simulink model "mat_model"  (R2013b)
settings: Solver=ode3  StartTime=0.0  StopTime=0.06  FixedStep=100e-6  RelTol=1e-3
undefined symbols (not defined in the file): E, f, L, L1, R, Ts
settings Model: Creator=sadzi  LastModifiedBy=sadzi
settings SolverCC: AlgebraicLoopSolver=LineSearch
settings ConfigurationSet: Description=SimMechanics 2G

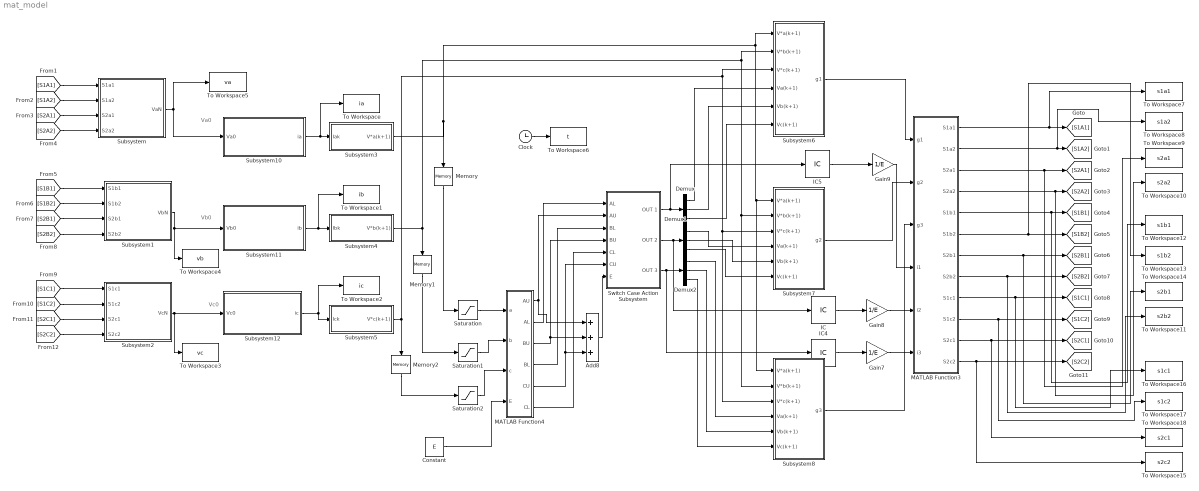
== system mat_model ==
  note: Vc0
  note: Va0
  note: Vb0
  Add8 : Sum  Inputs=+++
  Clock : Clock
  Constant : Constant  Value=E
  Demux : Demux  Outputs=3
  Demux1 : Demux  Outputs=3
  Demux2 : Demux  Outputs=3
  Gain7 : Gain  Gain=1/E
  Gain8 : Gain  Gain=1/E
  Gain9 : Gain  Gain=1/E
  IC : InitialCondition  Value=[0 0 0]
  IC4 : InitialCondition  Value=[0 0 0]
  IC5 : InitialCondition  Value=[0 0 0]
  MATLAB Function3 : MATLAB Function  TreatAsAtomicUnit=on
  MATLAB Function4 : MATLAB Function  TreatAsAtomicUnit=on
  Memory : Memory
  Memory1 : Memory
  Memory2 : Memory
  Saturation : Saturate  UpperLimit=2*E  LowerLimit=-2*E
  Saturation1 : Saturate  UpperLimit=2*E  LowerLimit=-2*E
  Saturation2 : Saturate  UpperLimit=2*E  LowerLimit=-2*E
  Subsystem : Subsystem
  Subsystem1 : Subsystem
  Subsystem10 : Subsystem
  Subsystem11 : Subsystem
  Subsystem12 : Subsystem
  Subsystem2 : Subsystem
  Subsystem3 : Subsystem
  Subsystem4 : Subsystem
  Subsystem5 : Subsystem
  Subsystem6 : Subsystem
  Subsystem7 : Subsystem
  Subsystem8 : Subsystem
  Switch Case Action Subsystem : Subsystem  TreatAsAtomicUnit=on
  To Workspace : ToWorkspace  VariableName=ia  SampleTime=-1
  To Workspace1 : ToWorkspace  VariableName=ib  SampleTime=-1
  To Workspace10 : ToWorkspace  VariableName=s2a2  SampleTime=-1
  To Workspace11 : ToWorkspace  VariableName=s2b2  SampleTime=-1
  To Workspace12 : ToWorkspace  VariableName=s1b1  SampleTime=-1
  To Workspace13 : ToWorkspace  VariableName=s1b2  SampleTime=-1
  To Workspace14 : ToWorkspace  VariableName=s2b1  SampleTime=-1
  To Workspace15 : ToWorkspace  VariableName=s2c2  SampleTime=-1
  To Workspace16 : ToWorkspace  VariableName=s1c1  SampleTime=-1
  To Workspace17 : ToWorkspace  VariableName=s1c2  SampleTime=-1
  To Workspace18 : ToWorkspace  VariableName=s2c1  SampleTime=-1
  To Workspace2 : ToWorkspace  VariableName=ic  SampleTime=-1
  To Workspace3 : ToWorkspace  VariableName=vc  SampleTime=-1
  To Workspace4 : ToWorkspace  VariableName=vb  SampleTime=-1
  To Workspace5 : ToWorkspace  VariableName=va  SampleTime=-1
  To Workspace6 : ToWorkspace  VariableName=t  SampleTime=-1
  To Workspace7 : ToWorkspace  VariableName=s1a1  SampleTime=-1
  To Workspace8 : ToWorkspace  VariableName=s1a2  SampleTime=-1
  To Workspace9 : ToWorkspace  VariableName=s2a1  SampleTime=-1
  wires:
  Subsystem/1(VaN) -> To Workspace5/1, Subsystem10/1(Va0)
  Subsystem3/1(V*a(k+1)) -> Subsystem8/1(V*a(k+1)), Subsystem7/1(V*a(k+1)), Subsystem6/1(V*a(k+1)), Memory/1
  Subsystem4/1(V*b(k+1)) -> Subsystem8/2(V*b(k+1)), Subsystem7/2(V*b(k+1)), Subsystem6/2(V*b(k+1)), Memory1/1
  Subsystem5/1(V*c(k+1)) -> Subsystem8/3(V*c(k+1)), Subsystem7/3(V*c(k+1)), Subsystem6/3(V*c(k+1)), Memory2/1
  MATLAB Function4/1(AU) -> Add8/1, Switch Case Action Subsystem/2(AU)
  MATLAB Function4/3(BU) -> Add8/2, Switch Case Action Subsystem/4(BU)
  MATLAB Function4/5(CU) -> Add8/3, Switch Case Action Subsystem/6(CU)
  MATLAB Function4/2(AL) -> Switch Case Action Subsystem/1(AL)
  MATLAB Function4/4(BL) -> Switch Case Action Subsystem/3(BL)
  MATLAB Function4/6(CL) -> Switch Case Action Subsystem/5(CL)
  Switch Case Action Subsystem/1(OUT 1) -> Demux/1, IC5/1
  Demux/1 -> Subsystem6/4(Va(k+1))
  Demux/2 -> Subsystem6/5(Vb(k+1))
  Demux/3 -> Subsystem6/6(Vc(k+1))
  Switch Case Action Subsystem/2(OUT 2) -> IC/1, Demux1/1
  Demux1/1 -> Subsystem7/4(Va(k+1))
  Demux1/2 -> Subsystem7/5(Vb(k+1))
  Demux1/3 -> Subsystem7/6(Vc(k+1))
  Switch Case Action Subsystem/3(OUT 3) -> IC4/1, Demux2/1
  Demux2/1 -> Subsystem8/4(Va(k+1))
  Demux2/2 -> Subsystem8/5(Vb(k+1))
  Demux2/3 -> Subsystem8/6(Vc(k+1))
  Subsystem1/1(VbN) -> To Workspace4/1, Subsystem11/1(Vb0)
  Subsystem2/1(VcN) -> To Workspace3/1, Subsystem12/1(Vc0)
  Subsystem7/1(g2) -> MATLAB Function3/2(g2)
  Subsystem6/1(g1) -> MATLAB Function3/1(g1)
  Subsystem8/1(g3) -> MATLAB Function3/3(g3)
  Saturation/1 -> MATLAB Function4/1(a)
  Saturation1/1 -> MATLAB Function4/2(b)
  Saturation2/1 -> MATLAB Function4/3(c)
  Add8/1 -> Switch Case Action Subsystem/7(E)
  Gain7/1 -> MATLAB Function3/6(i3)
  Gain8/1 -> MATLAB Function3/5(i2)
  Gain9/1 -> MATLAB Function3/4(i1)
  [S1A2] -> Subsystem/2(S1a2)
  [S2A1] -> Subsystem/3(S2a1)
  [S2A2] -> Subsystem/4(S2a2)
  [S1B1] -> Subsystem1/1(S1b1)
  [S1B2] -> Subsystem1/2(S1b2)
  [S2B1] -> Subsystem1/3(S2b1)
  [S2B2] -> Subsystem1/4(S2b2)
  [S1C1] -> Subsystem2/1(S1c1)
  [S1C2] -> Subsystem2/2(S1c2)
  [S2C1] -> Subsystem2/3(S2c1)
  [S2C2] -> Subsystem2/4(S2c2)
  [S1A1] -> Subsystem/1(S1a1)
  MATLAB Function3/1(S1a1) -> To Workspace7/1, [S1A1]
  IC/1 -> Gain8/1
  IC4/1 -> Gain7/1
  IC5/1 -> Gain9/1
  MATLAB Function3/2(S1a2) -> To Workspace8/1, [S1A2]
  MATLAB Function3/3(S2a1) -> To Workspace9/1, [S2A1]
  MATLAB Function3/4(S2a2) -> To Workspace10/1, [S2A2]
  MATLAB Function3/5(S1b1) -> To Workspace12/1, [S1B1]
  MATLAB Function3/6(S1b2) -> To Workspace13/1, [S1B2]
  MATLAB Function3/7(S2b1) -> To Workspace14/1, [S2B1]
  MATLAB Function3/8(S2b2) -> To Workspace11/1, [S2B2]
  MATLAB Function3/9(S1c1) -> To Workspace16/1, [S1C1]
  MATLAB Function3/10(S1c2) -> To Workspace17/1, [S1C2]
  MATLAB Function3/11(S2c1) -> To Workspace18/1, [S2C1]
  MATLAB Function3/12(S2c2) -> To Workspace15/1, [S2C2]
  Memory/1 -> Saturation/1
  Memory1/1 -> Saturation1/1
  Memory2/1 -> Saturation2/1
  Constant/1 -> MATLAB Function4/4(E)
  Subsystem10/1(ia) -> To Workspace/1, Subsystem3/1(Iak)
  Subsystem11/1(ib) -> To Workspace1/1, Subsystem4/1(Ibk)
  Subsystem12/1(ic) -> To Workspace2/1, Subsystem5/1(Ick)
  Clock/1 -> To Workspace6/1

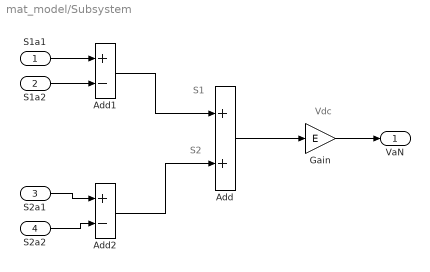
== system mat_model/Subsystem ==
  note: Vdc
  note: S2
  note: S1
  S1a1 : Inport
  S1a2 : Inport  Port=2
  S2a1 : Inport  Port=3
  S2a2 : Inport  Port=4
  Add : Sum
  Add1 : Sum  Inputs=+-
  Add2 : Sum  Inputs=+-
  Gain : Gain  Gain=E
  VaN : Outport
  wires:
  Add2/1 -> Add/2
  Add1/1 -> Add/1
  Add/1 -> Gain/1
  Gain/1 -> VaN/1
  S1a1/1 -> Add1/1
  S1a2/1 -> Add1/2
  S2a1/1 -> Add2/1
  S2a2/1 -> Add2/2

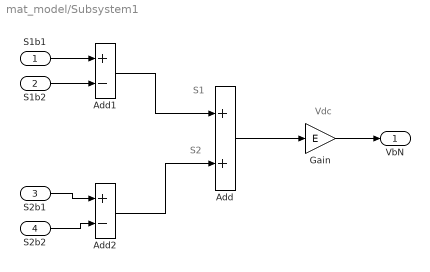
== system mat_model/Subsystem1 ==
  note: Vdc
  note: S2
  note: S1
  S1b1 : Inport
  S1b2 : Inport  Port=2
  S2b1 : Inport  Port=3
  S2b2 : Inport  Port=4
  Add : Sum
  Add1 : Sum  Inputs=+-
  Add2 : Sum  Inputs=+-
  Gain : Gain  Gain=E
  VbN : Outport
  wires:
  Add2/1 -> Add/2
  Add1/1 -> Add/1
  Add/1 -> Gain/1
  Gain/1 -> VbN/1
  S1b1/1 -> Add1/1
  S1b2/1 -> Add1/2
  S2b1/1 -> Add2/1
  S2b2/1 -> Add2/2

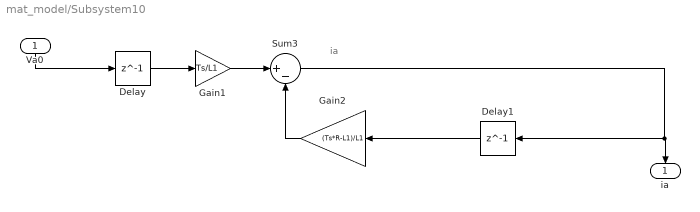
== system mat_model/Subsystem10 ==
  note: ia
  Va0 : Inport
  Delay : Delay  DelayLength=1  InitialCondition=0
  Delay1 : Delay  DelayLength=1  InitialCondition=0
  Gain1 : Gain  Gain=Ts/L1
  Gain2 : Gain  Gain=(Ts*R-L1)/L1
  Sum3 : Sum  Inputs=|+-
  ia : Outport
  wires:
  Delay/1 -> Gain1/1
  Gain1/1 -> Sum3/1
  Sum3/1 -> ia/1, Delay1/1
  Delay1/1 -> Gain2/1
  Gain2/1 -> Sum3/2
  Va0/1 -> Delay/1

== system mat_model/Subsystem11 ==
  note: ib
  Vb0 : Inport
  Delay2 : Delay  DelayLength=1  InitialCondition=0
  Delay3 : Delay  DelayLength=1  InitialCondition=0
  Gain3 : Gain  Gain=Ts/L
  Gain4 : Gain  Gain=(Ts*R-L)/L
  Sum1 : Sum  Inputs=|+-
  ib : Outport
  wires:
  Vb0/1 -> Delay2/1
  Delay2/1 -> Gain3/1
  Sum1/1 -> ib/1, Delay3/1
  Gain4/1 -> Sum1/2
  Gain3/1 -> Sum1/1
  Delay3/1 -> Gain4/1

== system mat_model/Subsystem12 ==
  note: ic
  Vc0 : Inport
  Delay4 : Delay  DelayLength=1  InitialCondition=0
  Delay5 : Delay  DelayLength=1  InitialCondition=0
  Gain5 : Gain  Gain=Ts/L
  Gain6 : Gain  Gain=(Ts*R-L)/L
  Sum2 : Sum  Inputs=|+-
  ic : Outport
  wires:
  Vc0/1 -> Delay4/1
  Delay4/1 -> Gain5/1
  Gain5/1 -> Sum2/1
  Delay5/1 -> Gain6/1
  Sum2/1 -> ic/1, Delay5/1
  Gain6/1 -> Sum2/2

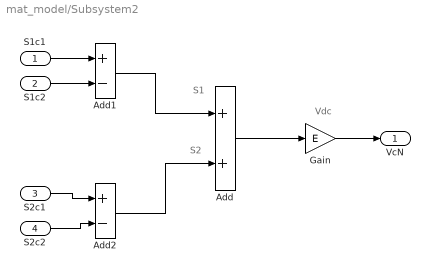
== system mat_model/Subsystem2 ==
  note: Vdc
  note: S2
  note: S1
  S1c1 : Inport
  S1c2 : Inport  Port=2
  S2c1 : Inport  Port=3
  S2c2 : Inport  Port=4
  Add : Sum
  Add1 : Sum  Inputs=+-
  Add2 : Sum  Inputs=+-
  Gain : Gain  Gain=E
  VcN : Outport
  wires:
  Add2/1 -> Add/2
  Add1/1 -> Add/1
  Add/1 -> Gain/1
  Gain/1 -> VcN/1
  S1c1/1 -> Add1/1
  S1c2/1 -> Add1/2
  S2c1/1 -> Add2/1
  S2c2/1 -> Add2/2

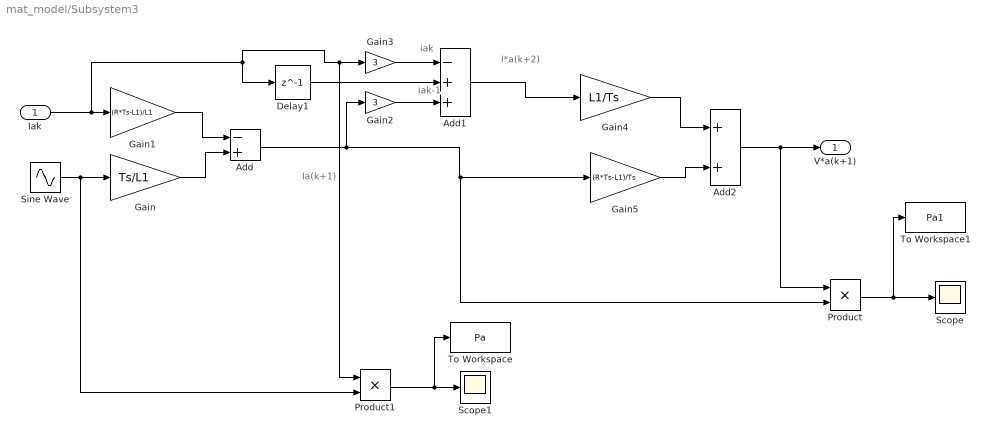
== system mat_model/Subsystem3 ==
  note: iak
  note: iak-1
  note: I*a(k+2)
  note: Ia(k+1)
  Iak : Inport
  Add : Sum  Inputs=-+
  Add1 : Sum  Inputs=-++
  Add2 : Sum
  Delay1 : Delay  DelayLength=1  InitialCondition=0
  Gain : Gain  Gain=Ts/L1
  Gain1 : Gain  Gain=(R*Ts-L1)/L1
  Gain2 : Gain  Gain=3
  Gain3 : Gain  Gain=3
  Gain4 : Gain  Gain=L1/Ts
  Gain5 : Gain  Gain=(R*Ts-L1)/Ts
  Product : Product
  Product1 : Product
  Scope : Scope
  Scope1 : Scope
  Sine Wave : Sin  SineType=Sample based  Amplitude=2*E  Frequency=f  Samples=spp  SampleTime=Ts
  To Workspace : ToWorkspace  VariableName=Pa  SampleTime=-1
  To Workspace1 : ToWorkspace  VariableName=Pa1  SampleTime=-1
  V*a(k+1) : Outport
  wires:
  Gain/1 -> Add/2
  Gain1/1 -> Add/1
  Add/1 -> Gain2/1, Product/2, Gain5/1
  Gain3/1 -> Add1/1
  Gain2/1 -> Add1/3
  Add1/1 -> Gain4/1
  Gain4/1 -> Add2/1
  Gain5/1 -> Add2/2
  Add2/1 -> Product/1, V*a(k+1)/1
  Sine Wave/1 -> Product1/2, Gain/1
  Delay1/1 -> Add1/2
  Product/1 -> To Workspace1/1, Scope/1
  Product1/1 -> To Workspace/1, Scope1/1
  Iak/1 -> Delay1/1, Product1/1, Gain3/1, Gain1/1

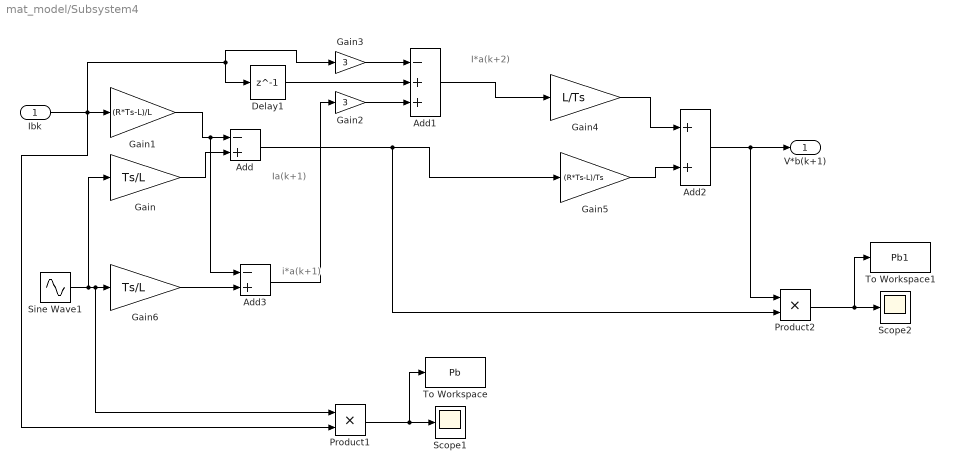
== system mat_model/Subsystem4 ==
  note: Ia(k+1)
  note: I*a(k+2)
  note: i*a(k+1)
  Ibk : Inport
  Add : Sum  Inputs=-+
  Add1 : Sum  Inputs=-++
  Add2 : Sum
  Add3 : Sum  Inputs=-+
  Delay1 : Delay  DelayLength=1  InitialCondition=0
  Gain : Gain  Gain=Ts/L
  Gain1 : Gain  Gain=(R*Ts-L)/L
  Gain2 : Gain  Gain=3
  Gain3 : Gain  Gain=3
  Gain4 : Gain  Gain=L/Ts
  Gain5 : Gain  Gain=(R*Ts-L)/Ts
  Gain6 : Gain  Gain=Ts/L
  Product1 : Product
  Product2 : Product
  Scope1 : Scope
      settings: SaveName=ScopeData2
  Scope2 : Scope
      settings: SaveName=ScopeData3
  Sine Wave1 : Sin  SineType=Sample based  Amplitude=2*E  Frequency=f  Phase=2.0943951  Samples=spp  SampleTime=Ts  Offset=nofs1
  To Workspace : ToWorkspace  VariableName=Pb  SampleTime=-1
  To Workspace1 : ToWorkspace  VariableName=Pb1  SampleTime=-1
  V*b(k+1) : Outport
  wires:
  Add2/1 -> Product2/1, V*b(k+1)/1
  Gain5/1 -> Add2/2
  Gain4/1 -> Add2/1
  Add1/1 -> Gain4/1
  Gain2/1 -> Add1/3
  Gain3/1 -> Add1/1
  Add/1 -> Product2/2, Gain5/1
  Gain/1 -> Add/2
  Sine Wave1/1 -> Gain/1, Product1/1, Gain6/1
  Gain1/1 -> Add3/1, Add/1
  Gain6/1 -> Add3/2
  Add3/1 -> Gain2/1
  Delay1/1 -> Add1/2
  Ibk/1 -> Gain3/1, Delay1/1, Product1/2, Gain1/1
  Product1/1 -> To Workspace/1, Scope1/1
  Product2/1 -> To Workspace1/1, Scope2/1

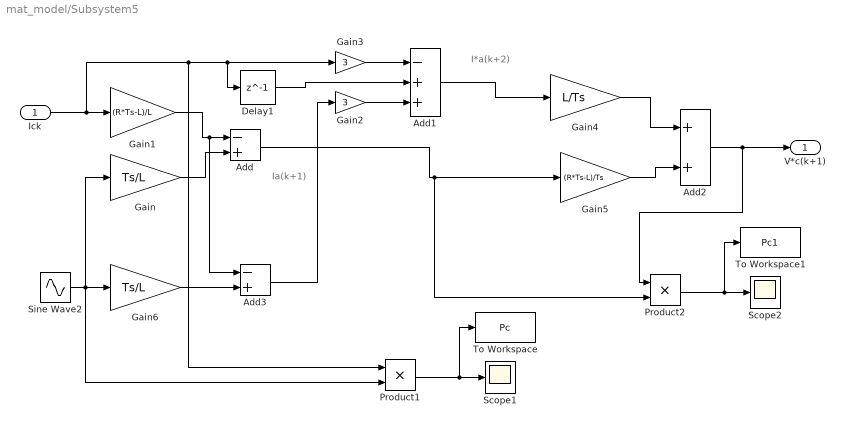
== system mat_model/Subsystem5 ==
  note: I*a(k+2)
  note: Ia(k+1)
  Ick : Inport
  Add : Sum  Inputs=-+
  Add1 : Sum  Inputs=-++
  Add2 : Sum
  Add3 : Sum  Inputs=-+
  Delay1 : Delay  DelayLength=1  InitialCondition=0
  Gain : Gain  Gain=Ts/L
  Gain1 : Gain  Gain=(R*Ts-L)/L
  Gain2 : Gain  Gain=3
  Gain3 : Gain  Gain=3
  Gain4 : Gain  Gain=L/Ts
  Gain5 : Gain  Gain=(R*Ts-L)/Ts
  Gain6 : Gain  Gain=Ts/L
  Product1 : Product
  Product2 : Product
  Scope1 : Scope
      settings: SaveName=ScopeData4
  Scope2 : Scope
      settings: SaveName=ScopeData5
  Sine Wave2 : Sin  SineType=Sample based  Amplitude=2*E  Frequency=f  Phase=4.1887902  Samples=spp  SampleTime=Ts  Offset=nofs2
  To Workspace : ToWorkspace  VariableName=Pc  SampleTime=-1
  To Workspace1 : ToWorkspace  VariableName=Pc1  SampleTime=-1
  V*c(k+1) : Outport
  wires:
  Gain/1 -> Add/2
  Add/1 -> Product2/2, Gain5/1
  Gain3/1 -> Add1/1
  Gain2/1 -> Add1/3
  Add1/1 -> Gain4/1
  Gain4/1 -> Add2/1
  Gain5/1 -> Add2/2
  Add2/1 -> Product2/1, V*c(k+1)/1
  Sine Wave2/1 -> Product1/2, Gain/1, Gain6/1
  Gain1/1 -> Add3/1, Add/1
  Gain6/1 -> Add3/2
  Add3/1 -> Gain2/1
  Delay1/1 -> Add1/2
  Ick/1 -> Product1/1, Delay1/1, Gain3/1, Gain1/1
  Product1/1 -> To Workspace/1, Scope1/1
  Product2/1 -> To Workspace1/1, Scope2/1

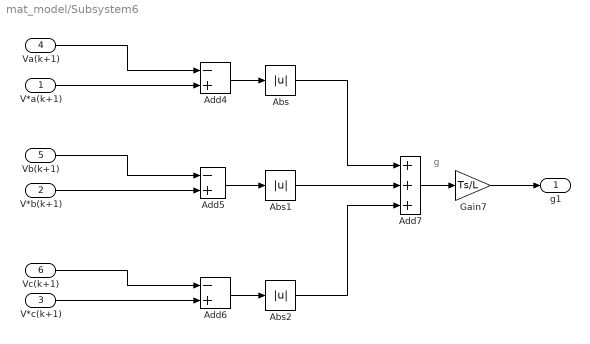
== system mat_model/Subsystem6 ==
  note: g
  V*a(k+1) : Inport
  V*b(k+1) : Inport  Port=2
  V*c(k+1) : Inport  Port=3
  Va(k+1) : Inport  Port=4
  Vb(k+1) : Inport  Port=5
  Vc(k+1) : Inport  Port=6
  Abs : Abs
  Abs1 : Abs
  Abs2 : Abs
  Add4 : Sum  Inputs=-+
  Add5 : Sum  Inputs=-+
  Add6 : Sum  Inputs=-+
  Add7 : Sum  Inputs=+++
  Gain7 : Gain  Gain=Ts/L
  g1 : Outport
  wires:
  V*a(k+1)/1 -> Add4/2
  Add4/1 -> Abs/1
  V*b(k+1)/1 -> Add5/2
  Add5/1 -> Abs1/1
  Vc(k+1)/1 -> Add6/1
  Add6/1 -> Abs2/1
  Abs1/1 -> Add7/2
  Abs/1 -> Add7/1
  Abs2/1 -> Add7/3
  Add7/1 -> Gain7/1
  Gain7/1 -> g1/1
  V*c(k+1)/1 -> Add6/2
  Vb(k+1)/1 -> Add5/1
  Va(k+1)/1 -> Add4/1

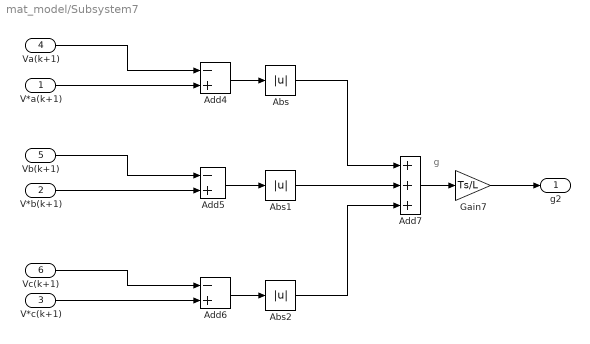
== system mat_model/Subsystem7 ==
  note: g
  V*a(k+1) : Inport
  V*b(k+1) : Inport  Port=2
  V*c(k+1) : Inport  Port=3
  Va(k+1) : Inport  Port=4
  Vb(k+1) : Inport  Port=5
  Vc(k+1) : Inport  Port=6
  Abs : Abs
  Abs1 : Abs
  Abs2 : Abs
  Add4 : Sum  Inputs=-+
  Add5 : Sum  Inputs=-+
  Add6 : Sum  Inputs=-+
  Add7 : Sum  Inputs=+++
  Gain7 : Gain  Gain=Ts/L
  g2 : Outport
  wires:
  Va(k+1)/1 -> Add4/1
  Vb(k+1)/1 -> Add5/1
  V*c(k+1)/1 -> Add6/2
  Gain7/1 -> g2/1
  Add7/1 -> Gain7/1
  Abs2/1 -> Add7/3
  Abs/1 -> Add7/1
  Abs1/1 -> Add7/2
  Add6/1 -> Abs2/1
  Vc(k+1)/1 -> Add6/1
  Add5/1 -> Abs1/1
  V*b(k+1)/1 -> Add5/2
  Add4/1 -> Abs/1
  V*a(k+1)/1 -> Add4/2

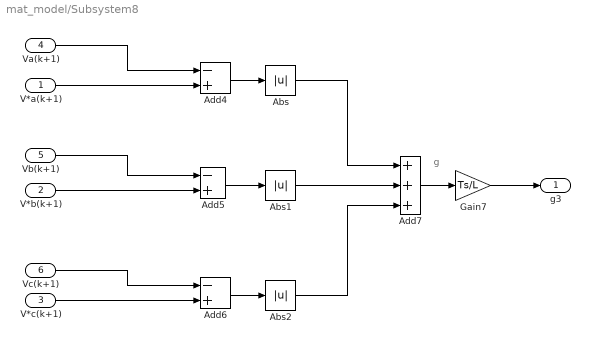
== system mat_model/Subsystem8 ==
  note: g
  V*a(k+1) : Inport
  V*b(k+1) : Inport  Port=2
  V*c(k+1) : Inport  Port=3
  Va(k+1) : Inport  Port=4
  Vb(k+1) : Inport  Port=5
  Vc(k+1) : Inport  Port=6
  Abs : Abs
  Abs1 : Abs
  Abs2 : Abs
  Add4 : Sum  Inputs=-+
  Add5 : Sum  Inputs=-+
  Add6 : Sum  Inputs=-+
  Add7 : Sum  Inputs=+++
  Gain7 : Gain  Gain=Ts/L
  g3 : Outport
  wires:
  V*a(k+1)/1 -> Add4/2
  Add4/1 -> Abs/1
  V*b(k+1)/1 -> Add5/2
  Add5/1 -> Abs1/1
  Vc(k+1)/1 -> Add6/1
  Add6/1 -> Abs2/1
  Abs1/1 -> Add7/2
  Abs/1 -> Add7/1
  Abs2/1 -> Add7/3
  Add7/1 -> Gain7/1
  Gain7/1 -> g3/1
  V*c(k+1)/1 -> Add6/2
  Vb(k+1)/1 -> Add5/1
  Va(k+1)/1 -> Add4/1

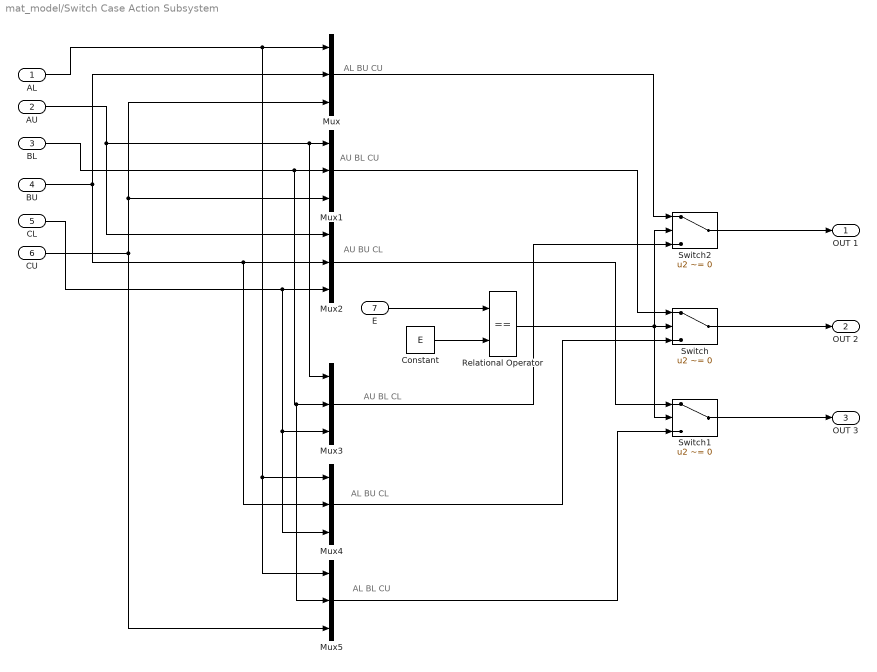
== system mat_model/Switch Case Action Subsystem ==
  note: AU BU CL
  note: AU BL CU
  note: AL BU CU
  note: AL BL CU
  note: AL BU CL
  note: AU BL CL
  AL : Inport
  AU : Inport  Port=2
  BL : Inport  Port=3
  BU : Inport  Port=4
  CL : Inport  Port=5
  CU : Inport  Port=6
  E : Inport  Port=7
  Constant : Constant  Value=E
  Mux{,1..5} (6 alike) : Mux  Inputs=3
  Relational Operator : RelationalOperator  Operator===  OutDataTypeStr=boolean
  Switch : Switch  Criteria=u2 ~= 0
  Switch1 : Switch  Criteria=u2 ~= 0
  Switch2 : Switch  Criteria=u2 ~= 0
  OUT 1 : Outport
  OUT 2 : Outport  Port=2
  OUT 3 : Outport  Port=3
  wires:
  AL/1 -> Mux5/1, Mux4/1, Mux/1
  BU/1 -> Mux4/2, Mux2/2, Mux/2
  AU/1 -> Mux2/1, Mux3/1, Mux1/1
  BL/1 -> Mux5/2, Mux3/2, Mux1/2
  CU/1 -> Mux5/3, Mux1/3, Mux/3
  CL/1 -> Mux4/3, Mux3/3, Mux2/3
  Constant/1 -> Relational Operator/2
  E/1 -> Relational Operator/1
  Relational Operator/1 -> Switch1/2, Switch2/2, Switch/2
  Mux3/1 -> Switch2/3
  Mux4/1 -> Switch/3
  Mux5/1 -> Switch1/3
  Mux/1 -> Switch2/1
  Mux1/1 -> Switch/1
  Mux2/1 -> Switch1/1
  Switch2/1 -> OUT 1/1
  Switch/1 -> OUT 2/1
  Switch1/1 -> OUT 3/1

== matlab function mat_model/MATLAB Function3 ==
  data: g1 input; S1a1 output; g2 input; g3 input; i1 input; S1a2 output; S2a1 output; S2a2 output; S1b1 output; S1b2 output; S2b1 output; S2b2 output; S1c1 output; S1c2 output; S2c1 output; S2c2 output; i2 input; i3 input
function [S1a1,S1a2,S2a1,S2a2,S1b1,S1b2,S2b1,S2b2,S1c1,S1c2,S2c1,S2c2] = fcn(g1,g2,g3,i1,i2,i3)
persistent s1a1 s1a2 s2a1 s2a2 s1b1 s1b2 s2b1 s2b2 s1c1 s1c2 s2c1 s2c2;

if isempty(s1a1)
    s1a1=0;
    s1a2=0;
    s2a1=0;
    s2a2=0;
    s1b1=0;
    s1b2=0;
    s2b1=0;
    s2b2=0;
    s1c1=0;
    s1c2=0;
    s2c1=0;
    s2c2=0;
end    
   
if(g1<=g2&&g1<=g3)
    [s11a,s12a,s21a,s22a]=signali(i1(1));
    [s11b,s12b,s21b,s22b]=signali(i1(2));
    [s11c,s12c,s21c,s22c]=signali(i1(3));
    s1a1=s11a;
    s1a2=s12a;
    s2a1=s21a;
    s2a2=s22a;
    s1b1=s11b;
    s1b2=s12b;
    s2b1=s21b;
    s2b2=s22b;
    s1c1=s11c;
    s1c2=s12c;
    s2c1=s21c;
    s2c2=s22c;
elseif(g2<=g1&&g2<=g3)
    [s11a,s12a,s21a,s22a]=signali(i2(1));
    [s11b,s12b,s21b,s22b]=signali(i2(2));
    [s11c,s12c,s21c,s22c]=signali(i2(3));
    s1a1=s11a;
    s1a2=s12a;
    s2a1=s21a;
    s2a2=s22a;
    s1b1=s11b;
    s1b2=s12b;
    s2b1=s21b;
    s2b2=s22b;
    s1c1=s11c;
    s1c2=s12c;
    s2c1=s21c;
    s2c2=s22c;
elseif(g3<=g1&&g3<=g2)
    [s11a,s12a,s21a,s22a]=signali(i3(1));
    [s11b,s12b,s21b,s22b]=signali(i3(2));
    [s11c,s12c,s21c,s22c]=signali(i3(3));
    s1a1=s11a;
    s1a2=s12a;
    s2a1=s21a;
    s2a2=s22a;
    s1b1=s11b;
    s1b2=s12b;
    s2b1=s21b;
    s2b2=s22b;
    s1c1=s11c;
    s1c2=s12c;
    s2c1=s21c;
    s2c2=s22c;
end





S1a1=s1a1;
S1a2=s1a2;
S2a1=s2a1;
S2a2=s2a2;
S1b1=s1b1;
S1b2=s1b2;
S2b1=s2b1;
S2b2=s2b2;
S1c1=s1c1;
S1c2=s1c2;
S2c1=s2c1;
S2c2=s2c2;

== matlab function mat_model/MATLAB Function4 ==
  data: a input; b input; AU output; AL output; BU output; BL output; c input; CU output; CL output; E input
function [AU,AL,BU,BL,CU,CL] = fcn(a,b,c,E)
persistent au al bu bl cu cl;
if isempty(au)
    au=0;
    bu=0;
    cu=0;
    al=0;
    bl=0;
    cl=0;
end

if(a<-E)
    if(b<0&&b>=-E)
        if(c>=E)
            au=-E; al=-2*E; bu=0; bl=-E; cu=2*E; cl=E;%1
        end
    elseif(b<E&&b>=0)
        if(c>=E)
            au=-E; al=-2*E; bu=E; bl=0; cu=2*E; cl=E;%2
        elseif(c<E&&c>=0)
            au=-E; al=-2*E; bu=E; bl=0; cu=E; cl=0;%3
        end
    elseif(b>=E)
        if(c<E&&c>=0)
            au=-E; al=-2*E; bu=2*E; bl=E; cu=E; cl=0;%4
        elseif(c<0&&c>=-E)
            au=-E; al=-2*E; bu=2*E; bl=E; cu=0; cl=-E;%5
        end
    end
    
    
elseif(a<0&&a>=-E)
    if(b<-E)
        if(c>=E)
            au=0; al=-E; bu=-E; bl=-2*E; cu=2*E; cl=E;%6
        end
    elseif(b<0&&b>=-E)
        if(c>=E)
            au=0; al=-E; bu=0; bl=-E; cu=2*E; cl=E;%7
        elseif(c<E&&c>=0)
            au=0; al=-E; bu=0; bl=-E; cu=E; cl=0;%8
        end
    elseif(b<E&&b>=0)
        if(c<E&&c>=0)
            au=0; al=-E; bu=E; bl=0; cu=E; cl=0;%9
        elseif(c<0&&c>=-E)
            au=0; al=-E; bu=E; bl=0; cu=0; cl=-E;%10
        end
    elseif(b>=E)
        if(c<0&&c>=-E)
            au=0; al=-E; bu=2*E; bl=E; cu=0; cl=-E;%11
        elseif(c<-E)
            au=0; al=-E; bu=2*E; bl=E; cu=-E; cl=-2*E;%12
        end
    end
    
    
elseif(a<E&&a>=0)
    if(b<-E)
        if(c>=E)
            au=E; al=0; bu=-E; bl=-2*E; cu=2*E; cl=E;%13
        elseif(c<E&&c>=0)
            au=E; al=0; bu=-E; bl=-2*E; cu=E; cl=0;%14
        end
    elseif(b<0&&b>=-E)
        if(c<E&&c>=0)
            au=E; al=0; bu=0; bl=-E; cu=E; cl=0;%15
        elseif(c<0&&c>=-E)
            au=E; al=0; bu=0; bl=-E; cu=0; cl=-E;%16
        end
    elseif(b<E&&b>=0)
        if(c<0&&c>=-E)
            au=E; al=0; bu=E; bl=0; cu=0; cl=-E;%17
        elseif(c<-E)
            au=E; al=0; bu=E; bl=0; cu=-E; cl=-2*E;%18
        end
    elseif(b>=E)
        if(c<=-E)
            au=E; al=0; bu=2*E; bl=E; cu=-E; cl=-2*E;%19
        end
    end
    
    
    
elseif(a>=E)
    if(b<-E)
        if(c<E&&c>=0)
            au=2*E; al=E; bu=-E; bl=-2*E; cu=E; cl=0;%20
        elseif(c<0&&c>=-E)
            au=2*E; al=E; bu=-E; bl=-2*E; cu=0; cl=-E;%21
        end
    elseif(b<0&&b>=-E)
        if(c<0&&c>=-E)
            au=2*E; al=E; bu=0; bl=-E; cu=0; cl=-E;%22
        elseif(c<-E)
            au=2*E; al=E; bu=0; bl=-E; cu=-E; cl=-2*E;%23
        end
    elseif(b<E&&b>=0)
        if(c<=-E)
            au=2*E; al=E; bu=E; bl=0; cu=-E; cl=-2*E;%24
        end
    end
    
    
end

% if(b<-E)
% elseif(b<0&&b>=-E)
% elseif(b<E&&b>=0)
% elseif(b>=E)
% end

AU=au;
BU=bu;
CU=cu;
AL=al;
BL=bl;
CL=cl;
